simulink library "DBX_Control_lib"  (R2015a)
settings: Solver=ode45  SolverMode=SingleTasking  StartTime=0.0  StopTime=10.0  RelTol=1e-3
undefined symbols (not defined in the file): a, A_M, C_d0, CG, h_1, h_2, h_3, hp_1, kappa_Q, kappa_T, L_M, lambda_0_Q, lambda_0_T, m, Newton, Omega_TO, R, Raphson, rho, Rotation_sign, sigma, T_ctrl, T_sim, theta_0, theta_1, Throtle_TO, Throtle_TTO_vec, v_i0, v_i_adim, Vx_adim, Vz_adim
libraries: DBX_Control_lib x15, vrlib x7, DBX_model x2, qcatlib x1, simulink x1, XXCopter_Control x1
(part 2 of 2)

== system DBX_Control_lib/Ref Model and PI Controller/PI Controller ==
  y_c : Inport
  y_meas : Inport  Port=2
  Anti-windup signal : Inport  Port=3
  Int_reset : Inport  Port=4
  " " : Sum  Inputs=++-
  " 1" : Sum  Inputs=|++
  Add : Sum  Inputs=|+-
  Discrete-Time Integrator : DiscreteIntegrator  ExternalReset=either  InitialConditionSetting=State (most efficient)  SampleTime=T_ctrl
  K_a : Gain  Gain=K_a
  K_b : Gain  Gain=K_b
  f_c : Gain  Gain=f_c
  f_i*K_b : Gain  Gain=f_i*K_b
  y_des_dot : Outport
  wires:
  f_i*K_b/1 -> " 1"/1
  Add/1 -> f_i*K_b/1
  K_b/1 -> y_des_dot/1
  y_meas/1 -> " "/3, Add/2
  y_c/1 -> f_c/1, Add/1
  Discrete-Time Integrator/1 -> " "/2
  f_c/1 -> " "/1
  " "/1 -> K_b/1
  Anti-windup signal/1 -> K_a/1
  " 1"/1 -> Discrete-Time Integrator/1
  K_a/1 -> " 1"/2
  Int_reset/1 -> Discrete-Time Integrator/2

== system DBX_Control_lib/Ref Model and PI Controller/Reference Model ==
  y_ref : Inport
  y_i : Inport  Port=2
  Int_reset : Inport  Port=3
  Add : Sum  Inputs=|+-
  Discrete-Time Integrator : DiscreteIntegrator  ExternalReset=either  InitialConditionSource=external  InitialConditionSetting=State (most efficient)  SampleTime=T_ctrl
  K_ref : Gain  Gain=1/tau
  y_c_dot : Outport
  y_c : Outport  Port=2
  wires:
  y_ref/1 -> Add/1
  Add/1 -> K_ref/1
  K_ref/1 -> y_c_dot/1, Discrete-Time Integrator/1
  Discrete-Time Integrator/1 -> Add/2, y_c/1
  y_i/1 -> Discrete-Time Integrator/3
  Int_reset/1 -> Discrete-Time Integrator/2

== system DBX_Control_lib/Arm Dynamics/Aerodynamics Propeller DBX/2D vec norm1 ==
  v : Inport
  norm^2rm : Subsystem  TreatAsAtomicUnit=on
  sqrt : Sqrt  AlgorithmType=Newton-Raphson  SaturateOnIntegerOverflow=on
  norm(v) : Outport
  wires:
  v/1 -> norm^2rm/1(v)
  norm^2rm/1(norm(v)) -> sqrt/1
  sqrt/1 -> norm(v)/1

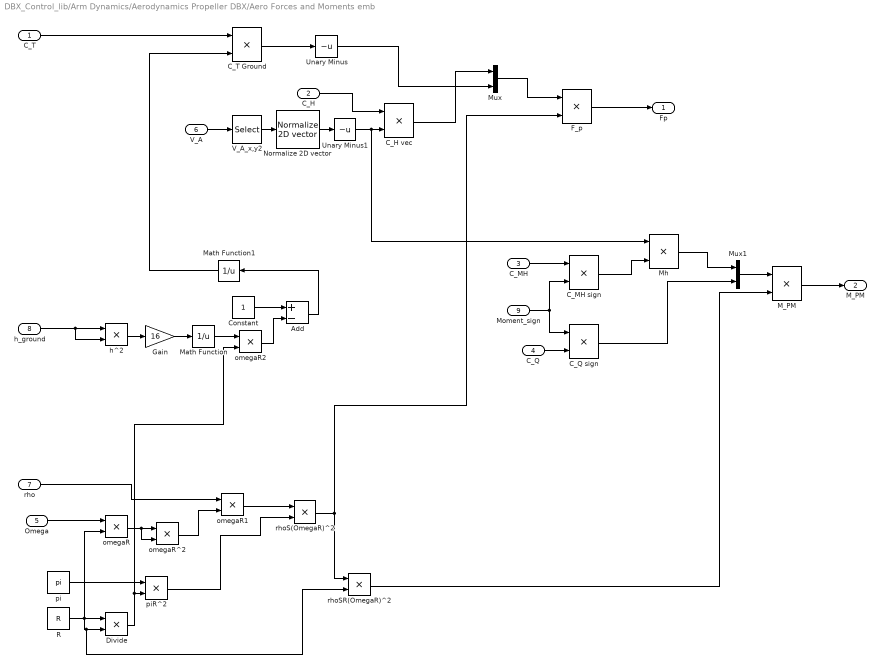
== system DBX_Control_lib/Arm Dynamics/Aerodynamics Propeller DBX/Aero Forces and Moments emb ==
  C_T : Inport
  C_H : Inport  Port=2
  C_MH : Inport  Port=3
  C_Q : Inport  Port=4
  Omega : Inport  Port=5
  V_A : Inport  Port=6
  rho : Inport  Port=7
  h_ground : Inport  Port=8
  Moment_sign : Inport  Port=9
  Add : Sum  Inputs=+-
  C_H vec : Product  Inputs=**
  C_MH sign : Product  Inputs=**
  C_Q sign : Product  Inputs=**
  C_T Ground : Product  Inputs=**
  Constant : Constant  OutDataTypeStr=single
  Divide : Product  Inputs=**
  F_p : Product  Inputs=**
  Gain : Gain  Gain=16  OutDataTypeStr=single
  M_PM : Product  Inputs=**
  Math Function : Math  Operator=reciprocal  SaturateOnIntegerOverflow=on
  Math Function1 : Math  Operator=reciprocal  SaturateOnIntegerOverflow=on
  Mh : Product  Inputs=**
  Mux : Mux  Inputs=[2,1]
  Mux1 : Mux  Inputs=[2,1]
  Normalize 2D vector : DBX_model/Normalize 2D vector
  R : Constant  Value=R  OutDataTypeStr=single
  Unary Minus : UnaryMinus
  Unary Minus1 : UnaryMinus
  V_A_x,y2 : Selector  IndexMode=Zero-based  InputPortWidth=3  Indices=[0,1]
  h^2 : Product  Inputs=**
  omegaR : Product  Inputs=**
  omegaR1 : Product  Inputs=**
  omegaR2 : Product  Inputs=**
  omegaR^2 : Product  Inputs=**
  pi : Constant  Value=pi  OutDataTypeStr=single
  piR^2 : Product  Inputs=**
  rhoS(OmegaR)^2 : Product  Inputs=**
  rhoSR(OmegaR)^2 : Product  Inputs=**
  Fp : Outport
  "M_PM " : Outport  Port=2
  wires:
  M_PM/1 -> "M_PM "/1
  rhoSR(OmegaR)^2/1 -> M_PM/2
  C_Q sign/1 -> Mux1/2
  C_Q/1 -> C_Q sign/2
  Mux1/1 -> M_PM/1
  F_p/1 -> Fp/1
  Mh/1 -> Mux1/1
  C_MH sign/1 -> Mh/2
  Moment_sign/1 -> C_Q sign/1, C_MH sign/2
  C_MH/1 -> C_MH sign/1
  rhoS(OmegaR)^2/1 -> F_p/2, rhoSR(OmegaR)^2/1
  Mux/1 -> F_p/1
  Unary Minus/1 -> Mux/2
  C_H vec/1 -> Mux/1
  C_H/1 -> C_H vec/1
  Unary Minus1/1 -> C_H vec/2, Mh/1
  Normalize 2D vector/1 -> Unary Minus1/1
  V_A/1 -> V_A_x,y2/1
  V_A_x,y2/1 -> Normalize 2D vector/1
  C_T Ground/1 -> Unary Minus/1
  Math Function1/1 -> C_T Ground/2
  Add/1 -> Math Function1/1
  omegaR2/1 -> Add/2
  Constant/1 -> Add/1
  Math Function/1 -> omegaR2/1
  Gain/1 -> Math Function/1
  h^2/1 -> Gain/1
  h_ground/1 -> h^2/1, h^2/2
  C_T/1 -> C_T Ground/1
  omegaR1/1 -> rhoS(OmegaR)^2/1
  piR^2/1 -> rhoS(OmegaR)^2/2
  omegaR^2/1 -> omegaR1/2
  omegaR/1 -> omegaR^2/1, omegaR^2/2
  rho/1 -> omegaR1/1
  Omega/1 -> omegaR/1
  Divide/1 -> piR^2/2, omegaR2/2
  pi/1 -> piR^2/1
  R/1 -> Divide/1, omegaR/2, Divide/2, rhoSR(OmegaR)^2/2

== system DBX_Control_lib/Arm Dynamics/Aerodynamics Propeller DBX/RAND_induced ==
  v_x_adim : Inport
  v_z_adim : Inport  Port=2
  Constant : Constant  OutDataTypeStr=single
  Divide : Product  Inputs=*/
  If : If  IfExpression=u1<=-2  ElseIfExpressions=u1>-2 & u1<0, u1 >= 0  ShowElse=off
  If Action Subsystem : Subsystem  TreatAsAtomicUnit=on
  If Action Subsystem1 : Subsystem  TreatAsAtomicUnit=on
  If Action Subsystem2 : Subsystem  TreatAsAtomicUnit=on
  Math Function : Math  Operator=square  SaturateOnIntegerOverflow=on
  Merge : Merge  Inputs=3
  Sqrt : Sqrt  SaturateOnIntegerOverflow=on
  Sum : Sum  Inputs=|++
  v_i_adim : Outport
  wires:
  Divide/1 -> v_i_adim/1
  Sqrt/1 -> Divide/2
  v_x_adim/1 -> Math Function/1, If/1
  Sum/1 -> Sqrt/1
  If/3 -> If Action Subsystem2/Action
  If/2 -> If Action Subsystem1/Action
  Constant/1 -> Sum/2
  Math Function/1 -> Sum/1
  v_z_adim/1 -> If Action Subsystem2/1(In1), If Action Subsystem1/1(v_z_adim), If Action Subsystem/1(v_z_adim)
  Merge/1 -> Divide/1
  If Action Subsystem2/1(Out1) -> Merge/3
  If Action Subsystem1/1(v_ia_adim) -> Merge/2
  If Action Subsystem/1(v_ia_adim) -> Merge/1
  If/1 -> If Action Subsystem/Action

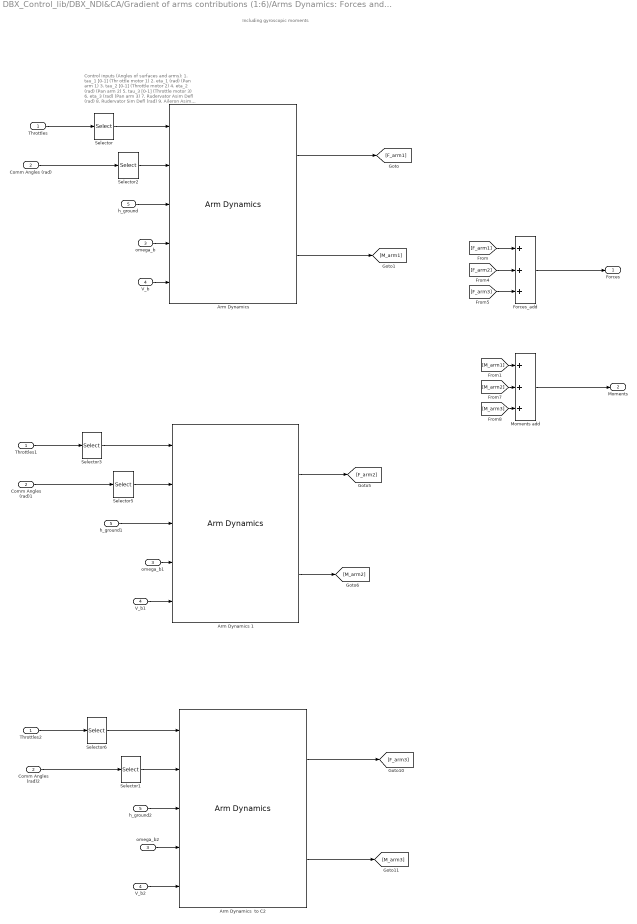
== system DBX_Control_lib/DBX_NDI&CA/Gradient of arms contributions (1:6)/Arms Dynamics: Forces and Moments ==
  note: Control inputs (Angles  of surfaces and arms):
      |
      | 1. tau_1 [0-1] (Thr ottle motor 1)
      | 2. eta_1 (rad)  (Pan arm 1)
      |
      | 3. tau_2 [0-1] (Throttle motor 2)
      | 4. eta_2 (rad)  (Pan arm 2)
      |
      | 5. tau_3 [0-1] (Throttle motor 3)
      | 6. eta_3 (rad)  (Pan arm  3)
      |
      | 7. Rudervator Asim Defl (rad)
      | 8. Rudervator Sim Defl (rad)
      | 9. Aileron Asim Defl (rad)
  note: Including gyroscopic moments
  Throttles : Inport
  Comm Angles (rad) : Inport  Port=2
  omega_b : Inport  Port=3
  V_b : Inport  Port=4
  h_ground : Inport  Port=5
  "Arm Dynamics " : DBX_Control_lib/Arm Dynamics  arm_num=1  Rot_sign=Rotation_sign(1)  Hub_pos=[1/3*L_M;-A_M/2;h_1]  h_p=hp_1
  Arm Dynamics  to C2 : DBX_Control_lib/Arm Dynamics  arm_num=3  Rot_sign=Rotation_sign(3)  Hub_pos=[-2/3*L_M;0;h_3]  h_p=hp_3
  Arm Dynamics 1 : DBX_Control_lib/Arm Dynamics  arm_num=2  Rot_sign=Rotation_sign(2)  Hub_pos=[1/3*L_M;A_M/2;h_2]  h_p=hp_2
  Comm Angles (rad)1 : InportShadow  Port=2
  Comm Angles (rad)2 : InportShadow  Port=2
  Forces_add : Sum  Inputs=+++
  Moments add : Sum  Inputs=+++
  Selector : Selector  IndexMode=Zero-based  InputPortWidth=3  Indices=0
  Selector1 : Selector  IndexMode=Zero-based  InputPortWidth=3  Indices=2
  Selector2 : Selector  InputPortWidth=3
  Selector3 : Selector  IndexMode=Zero-based  InputPortWidth=3
  Selector5 : Selector  InputPortWidth=3  Indices=2
  Selector6 : Selector  IndexMode=Zero-based  InputPortWidth=3  Indices=2
  Throttles1 : InportShadow
  Throttles2 : InportShadow
  V_b1 : InportShadow  Port=4
  V_b2 : InportShadow  Port=4
  h_ground1 : InportShadow  Port=5
  h_ground2 : InportShadow  Port=5
  omega_b1 : InportShadow  Port=3
  omega_b2 : InportShadow  Port=3
  Forces : Outport
  Moments : Outport  Port=2
  wires:
  V_b2/1 -> Arm Dynamics  to C2/5
  Arm Dynamics 1/2 -> [M_arm2]
  Throttles/1 -> Selector/1
  Selector/1 -> "Arm Dynamics "/1
  V_b/1 -> "Arm Dynamics "/5
  Forces_add/1 -> Forces/1
  Moments add/1 -> Moments/1
  h_ground/1 -> "Arm Dynamics "/3
  "Arm Dynamics "/1 -> [F_arm1]
  "Arm Dynamics "/2 -> [M_arm1]
  [F_arm1] -> Forces_add/1
  [M_arm1] -> Moments add/1
  omega_b/1 -> "Arm Dynamics "/4
  [F_arm2] -> Forces_add/2
  [F_arm3] -> Forces_add/3
  [M_arm3] -> Moments add/3
  [M_arm2] -> Moments add/2
  Selector2/1 -> "Arm Dynamics "/2
  Comm Angles (rad)/1 -> Selector2/1
  Throttles1/1 -> Selector3/1
  Selector3/1 -> Arm Dynamics 1/1
  V_b1/1 -> Arm Dynamics 1/5
  h_ground1/1 -> Arm Dynamics 1/3
  omega_b1/1 -> Arm Dynamics 1/4
  Selector5/1 -> Arm Dynamics 1/2
  Comm Angles (rad)1/1 -> Selector5/1
  Throttles2/1 -> Selector6/1
  Selector6/1 -> Arm Dynamics  to C2/1
  h_ground2/1 -> Arm Dynamics  to C2/3
  Arm Dynamics  to C2/1 -> [F_arm3]
  Arm Dynamics  to C2/2 -> [M_arm3]
  omega_b2/1 -> Arm Dynamics  to C2/4
  Selector1/1 -> Arm Dynamics  to C2/2
  Comm Angles (rad)2/1 -> Selector1/1
  Arm Dynamics 1/1 -> [F_arm2]

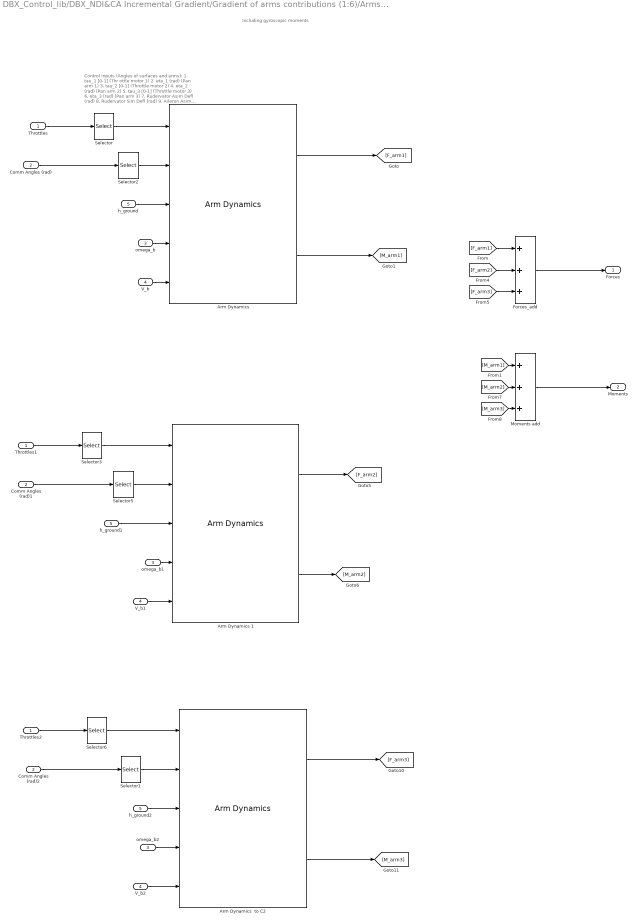
== system DBX_Control_lib/DBX_NDI&CA Incremental Gradient/Gradient of arms contributions (1:6)/Arms Dynamics: Forces and Moments ==
  note: Control inputs (Angles  of surfaces and arms):
      |
      | 1. tau_1 [0-1] (Thr ottle motor 1)
      | 2. eta_1 (rad)  (Pan arm 1)
      |
      | 3. tau_2 [0-1] (Throttle motor 2)
      | 4. eta_2 (rad)  (Pan arm 2)
      |
      | 5. tau_3 [0-1] (Throttle motor 3)
      | 6. eta_3 (rad)  (Pan arm  3)
      |
      | 7. Rudervator Asim Defl (rad)
      | 8. Rudervator Sim Defl (rad)
      | 9. Aileron Asim Defl (rad)
  note: Including gyroscopic moments
  Throttles : Inport
  Comm Angles (rad) : Inport  Port=2
  omega_b : Inport  Port=3
  V_b : Inport  Port=4
  h_ground : Inport  Port=5
  "Arm Dynamics " : DBX_Control_lib/Arm Dynamics  arm_num=1  Rot_sign=Rotation_sign(1)  Hub_pos=[1/3*L_M;-A_M/2;h_1]  h_p=hp_1
  Arm Dynamics  to C2 : DBX_Control_lib/Arm Dynamics  arm_num=3  Rot_sign=Rotation_sign(3)  Hub_pos=[-2/3*L_M;0;h_3]  h_p=hp_3
  Arm Dynamics 1 : DBX_Control_lib/Arm Dynamics  arm_num=2  Rot_sign=Rotation_sign(2)  Hub_pos=[1/3*L_M;A_M/2;h_2]  h_p=hp_2
  Comm Angles (rad)1 : InportShadow  Port=2
  Comm Angles (rad)2 : InportShadow  Port=2
  Forces_add : Sum  Inputs=+++
  Moments add : Sum  Inputs=+++
  Selector : Selector  IndexMode=Zero-based  InputPortWidth=3  Indices=0
  Selector1 : Selector  IndexMode=Zero-based  InputPortWidth=3  Indices=2
  Selector2 : Selector  InputPortWidth=3
  Selector3 : Selector  IndexMode=Zero-based  InputPortWidth=3
  Selector5 : Selector  InputPortWidth=3  Indices=2
  Selector6 : Selector  IndexMode=Zero-based  InputPortWidth=3  Indices=2
  Throttles1 : InportShadow
  Throttles2 : InportShadow
  V_b1 : InportShadow  Port=4
  V_b2 : InportShadow  Port=4
  h_ground1 : InportShadow  Port=5
  h_ground2 : InportShadow  Port=5
  omega_b1 : InportShadow  Port=3
  omega_b2 : InportShadow  Port=3
  Forces : Outport
  Moments : Outport  Port=2
  wires:
  V_b2/1 -> Arm Dynamics  to C2/5
  Arm Dynamics 1/2 -> [M_arm2]
  Throttles/1 -> Selector/1
  Selector/1 -> "Arm Dynamics "/1
  V_b/1 -> "Arm Dynamics "/5
  Forces_add/1 -> Forces/1
  Moments add/1 -> Moments/1
  h_ground/1 -> "Arm Dynamics "/3
  "Arm Dynamics "/1 -> [F_arm1]
  "Arm Dynamics "/2 -> [M_arm1]
  [F_arm1] -> Forces_add/1
  [M_arm1] -> Moments add/1
  omega_b/1 -> "Arm Dynamics "/4
  [F_arm2] -> Forces_add/2
  [F_arm3] -> Forces_add/3
  [M_arm3] -> Moments add/3
  [M_arm2] -> Moments add/2
  Selector2/1 -> "Arm Dynamics "/2
  Comm Angles (rad)/1 -> Selector2/1
  Throttles1/1 -> Selector3/1
  Selector3/1 -> Arm Dynamics 1/1
  V_b1/1 -> Arm Dynamics 1/5
  h_ground1/1 -> Arm Dynamics 1/3
  omega_b1/1 -> Arm Dynamics 1/4
  Selector5/1 -> Arm Dynamics 1/2
  Comm Angles (rad)1/1 -> Selector5/1
  Throttles2/1 -> Selector6/1
  Selector6/1 -> Arm Dynamics  to C2/1
  h_ground2/1 -> Arm Dynamics  to C2/3
  Arm Dynamics  to C2/1 -> [F_arm3]
  Arm Dynamics  to C2/2 -> [M_arm3]
  omega_b2/1 -> Arm Dynamics  to C2/4
  Selector1/1 -> Arm Dynamics  to C2/2
  Comm Angles (rad)2/1 -> Selector1/1
  Arm Dynamics 1/1 -> [F_arm2]

== system DBX_Control_lib/Normalize 4D vector/4D vec norm/norm^2rm ==
  v : Inport
  Demux : Demux
  Product{,1..3} (4 alike) : Product
  Sum : Sum  Inputs=4
  norm(v) : Outport
  wires:
  Product3/1 -> Sum/4
  Demux/4 -> Product3/1, Product3/2
  Product2/1 -> Sum/3
  Demux/3 -> Product2/1, Product2/2
  v/1 -> Demux/1
  Sum/1 -> norm(v)/1
  Product/1 -> Sum/1
  Product1/1 -> Sum/2
  Demux/1 -> Product/1, Product/2
  Demux/2 -> Product1/1, Product1/2

== system DBX_Control_lib/Arm Dynamics/Aerodynamics Propeller DBX/2D vec norm1/norm^2rm ==
  v : Inport
  Demux : Demux  Outputs=2
  Product : Product
  Product1 : Product
  Sum : Sum  Inputs=2
  norm(v) : Outport
  wires:
  Demux/1 -> Product/1, Product/2
  Product1/1 -> Sum/2
  Product/1 -> Sum/1
  Sum/1 -> norm(v)/1
  v/1 -> Demux/1
  Demux/2 -> Product1/2, Product1/1

== system DBX_Control_lib/Arm Dynamics/Aerodynamics Propeller DBX/RAND_induced/If Action Subsystem ==
  v_z_adim : Inport
  Action Port : ActionPort
  Subsystem : Subsystem
  v_ia_adim : Outport
  wires:
  v_z_adim/1 -> Subsystem/1(v_z_adim)
  Subsystem/1(v_ia_adim #1) -> v_ia_adim/1

== system DBX_Control_lib/Arm Dynamics/Aerodynamics Propeller DBX/RAND_induced/If Action Subsystem1 ==
  v_z_adim : Inport
  Action Port : ActionPort
  Subsystem1 : Subsystem
  v_ia_adim : Outport
  wires:
  v_z_adim/1 -> Subsystem1/1(v_z_adim)
  Subsystem1/1(v_ia_adim #2) -> v_ia_adim/1

== system DBX_Control_lib/Arm Dynamics/Aerodynamics Propeller DBX/RAND_induced/If Action Subsystem2 ==
  In1 : Inport
  Action Port : ActionPort
  Subsystem1 : Subsystem
  Out1 : Outport
  wires:
  In1/1 -> Subsystem1/1(v_z_adim)
  Subsystem1/1(v_ia_adim #3) -> Out1/1

== system DBX_Control_lib/Arm Dynamics/Aerodynamics Propeller DBX/RAND_induced/If Action Subsystem/Subsystem ==
  v_z_adim : Inport
  Constant1 : Constant  Value=4  OutDataTypeStr=single
  Gain : Gain  Gain=0.5  OutDataTypeStr=single
  Math Function : Math  Operator=square  SaturateOnIntegerOverflow=on
  Sqrt1 : Sqrt  SaturateOnIntegerOverflow=on
  Sum : Sum  Inputs=|++
  Sum1 : Sum  Inputs=|+-
  Unary Minus : UnaryMinus
  v_ia_adim #1 : Outport
  wires:
  Gain/1 -> Unary Minus/1
  Unary Minus/1 -> v_ia_adim #1/1
  Math Function/1 -> Sum1/1
  Constant1/1 -> Sum1/2
  Sum1/1 -> Sqrt1/1
  v_z_adim/1 -> Math Function/1, Sum/1
  Sum/1 -> Gain/1
  Sqrt1/1 -> Sum/2

== system DBX_Control_lib/Arm Dynamics/Aerodynamics Propeller DBX/RAND_induced/If Action Subsystem1/Subsystem1 ==
  v_z_adim : Inport
  25/12 : Constant  Value=2.083333333333334  OutDataTypeStr=single
  "3 " : Constant  Value=3  OutDataTypeStr=single
  7/6 : Constant  Value=1.166666666666667  OutDataTypeStr=single
  Constant1 : Constant  OutDataTypeStr=single
  Gain : Gain  Gain=0.5  OutDataTypeStr=single
  Math Function : Math  Operator=pow  SaturateOnIntegerOverflow=on
  Multiply : Product  Inputs=**
  Multiply1 : Product  Inputs=**
  Sum : Sum  Inputs=+-++
  v_ia_adim #2 : Outport
  wires:
  v_z_adim/1 -> Gain/1, Math Function/1, Multiply/1
  Sum/1 -> v_ia_adim #2/1
  25/12/1 -> Multiply/2
  Gain/1 -> Sum/2
  Constant1/1 -> Sum/1
  Multiply/1 -> Sum/3
  "3 "/1 -> Math Function/2
  Math Function/1 -> Multiply1/1
  7/6/1 -> Multiply1/2
  Multiply1/1 -> Sum/4

== system DBX_Control_lib/Arm Dynamics/Aerodynamics Propeller DBX/RAND_induced/If Action Subsystem2/Subsystem1 ==
  v_z_adim : Inport
  1 : Constant  Value=4  OutDataTypeStr=single
  Gain1 : Gain  Gain=0.5  OutDataTypeStr=single
  Math Function : Math  Operator=square  SaturateOnIntegerOverflow=on
  Sqrt : Sqrt  SaturateOnIntegerOverflow=on
  Sum : Sum  Inputs=|++
  Sum1 : Sum  Inputs=-+
  v_ia_adim #3 : Outport
  wires:
  Gain1/1 -> v_ia_adim #3/1
  Sum1/1 -> Gain1/1
  v_z_adim/1 -> Math Function/1, Sum1/1
  1/1 -> Sum/2
  Sum/1 -> Sqrt/1
  Math Function/1 -> Sum/1
  Sqrt/1 -> Sum1/2

== matlab function DBX_Control_lib/Arm Dynamics/Aerodynamics Propeller DBX/Prop Coefficients MOD ==
  data: lambda input; C_T output; mu input; C_H output; C_MH output; C_Q output; sigma parameter; C_d0 parameter; a parameter; theta_0 parameter; theta_1 parameter; lambda_0_T parameter; kappa_T parameter; lambda_0_Q parameter; kappa_Q parameter
function [C_T,C_H,C_MH,C_Q] = Aero_coeff_MOD(lambda,mu, sigma, C_d0, a, theta_0, theta_1,lambda_0_T,kappa_T,lambda_0_Q,kappa_Q)

C_T = sigma*a/4*(theta_0*(2/3+mu^2) +theta_1/2*(1+mu^2) -  kappa_T*(lambda-lambda_0_T)^2 );
C_Q =    +sigma*a/4*( 2/3*theta_0 -  kappa_Q*(lambda-lambda_0_Q)^2  + theta_1/2)*kappa_Q*(lambda-lambda_0_Q)^2 + sigma*C_d0/8*(1+mu^2);   % Always positive!!!


C_H= sigma*a/4*mu*lambda*(theta_0+theta_1/2) + sigma*C_d0/4*mu; 
C_MH= sigma*a/4*( 2/3*theta_0*mu-1/2*lambda*mu+theta_1*mu/2  );

== matlab function DBX_Control_lib/Arm Dynamics/Arms Kinematics DBX/DCM Arm ==
  data: arm_no input; eta input; T_Fb_FA output
function T_Fb_FA = DCM_Arm(arm_no,eta)
if arm_no==1 || arm_no==2
    T_Fb_FA = [ cos(eta),0,-sin(eta);
                    0,1,0;
                sin(eta),0,cos(eta)];
elseif arm_no==3 
    T_Fb_FA = [1,0,0;
                0,cos(eta),sin(eta);
                0,-sin(eta),cos(eta)];
else
    error('That is not right: Chose a right arm'); 
end

== matlab function DBX_Control_lib/DBX_NDI&CA Incremental Gradient/Get gradient ==
  data: index input; epsilon input; CA_Grad output; Perturb_evaluations input; CA_Grad_ant input
function CA_Grad  = Get_gradient(index, epsilon,Perturb_evaluations,CA_Grad_ant)

CA_Grad = CA_Grad_ant;

% Gradient of Arms: update
CA_Grad(:,index)= ( Perturb_evaluations(:,2)-Perturb_evaluations(:,1)  )./(epsilon);


% Eliminar componentes irrelevantes por el momento
CA_Grad(:,2)=zeros(6,1);
CA_Grad(:,4)=zeros(6,1);
CA_Grad(end,5)=0;
%% Add here the gradient of aerodynamics

% CA_Grad(4:6,7:10) ,,  B_adim*1/2*rho*S_w*TAS^2?? Cambiar esto esta mal


end

== matlab function DBX_Control_lib/Control allocator 4 coder/Embedded MATLAB Function ==
  data: v input; u output size=[9,1]; u_ant input; W input; ud input; B input; plim input; rlim input; T input size=1; Wv input; Wu input; gammma input size=1; imax input; W_out output size=[9,1]
function [u , W_out ] = qp_ca_WLS(v,u_ant,W,ud,B,plim,rlim,T,Wv,Wu, gammma,imax)


% Formulate as a regular QP problem: min ||Wu(u-ud)||

% Overall position limits
if isempty(rlim)
    umin = plim(:,1);
    umax = plim(:,2);
else
    umin = max(plim(:,1),u_ant+rlim(:,1)*T);
    umax = min(plim(:,2),u_ant+rlim(:,2)*T);
end

% Start with the last
u=u_ant;
W_out=W;

% Number of variables
m = length(umin);
%   Wu*(u-ud)
% Set default values of optional arguments
if nargin < 11
    imax = 100; % Heuristic value
    [k,m] = size(B);
    if nargin < 10, u = (umin+umax)/2; W = zeros(m,1); end
    if nargin < 8,  gammma = 1e6;       end
    if nargin < 7,  ud = zeros(m,1); end
    if nargin < 6,  Wu = eye(m);     end
    if nargin < 5,  Wv = eye(k);     end
end

gammma_sq = sqrt(gammma);
A = [gammma_sq*Wv*B ; Wu];
b = [gammma_sq*Wv*v ; Wu*ud];

% Initial residual.
d = b - A*u;
% Determine indeces of free variables.
i_free = zeros(size(W));
i_free = (W==0);

% Iterate until optimum is found or maximum number of iterations
% is reached.
for iter = 1:imax
    % ----------------------------------------
    %  Compute optimal perturbation vector p.
    % ----------------------------------------
    
    % Eliminate saturated variables.
    A_free = A(:,i_free);
    % Solve the reduced optimization problem for free variables.
    p_free = A_free\d;
    % Zero all perturbations corresponding to active constraints.
    p = zeros(m,1);
    % Insert perturbations from p_free into free the variables.
    p(i_free) = p_free;
    
    % ----------------------------
    %  Is the new point feasible?
    % ----------------------------
    
    u_opt = u + p;
    infeasible = (u_opt < umin) | (u_opt > umax);
    
    if ~any(infeasible(i_free))
        
        % ----------------------------
        %  Yes, check for optimality.
        % ----------------------------
        
        % Update point and residual.
        u = u_opt;
        d = d - A_free*p_free;
        % Compute Lagrangian multipliers.
        lambda = W.*(A'*d);
        % Are all lambda non-negative?
        if min(lambda) >= -eps
            % / ------------------------ \
            % | Optimum found, bail out. |
            % \ ------------------------ /
            return;
        end
        
        % --------------------------------------------------
        %  Optimum not found, remove one active constraint.
        % --------------------------------------------------
        
        % Remove constraint with most negative lambda from the
        % working set.
        [lambda_neg,i_neg] = min(lambda);
        W_out(i_neg) = 0;
        i_free(i_neg) = 1;
        
    else
        
        % ---------------------------------------
        %  No, find primary bounding constraint.
        % ---------------------------------------
        
        % Compute distances to the different boundaries. Since alpha < 1
        % is the maximum step length, initiate with ones.
        dist = ones(m,1);
        i_min = i_free & p<0;
        i_max = i_free & p>0;
        
        dist(i_min) = (umin(i_min) - u(i_min)) ./ p(i_min);
        dist(i_max) = (umax(i_max) - u(i_max)) ./ p(i_max);
        
        % Proportion of p to travel
        [alpha,i_alpha] = min(dist);
        % Update point and residual.
        u = u + alpha*p;
        d = d - A_free*alpha*p_free;
        
        % Add corresponding constraint to working set.
        W_out(i_alpha) = sign(p(i_alpha));
        i_free(i_alpha) = 0;
        
    end
    
    
end


end

== matlab function DBX_Control_lib/DBX_NDI&CA/Gravity Force and Moment ==
  data: q input; F_g_b output; M_g_b output; mass input; CG input; g parameter
function [F_g_b,M_g_b]   = Grav_Forces_and_Mom( q,mass,CG, g)

Prod=HamiltonProduct([q(1);-q(2);-q(3);-q(4)],HamiltonProduct([0;0;0;mass*g],[q(1);q(2);q(3);q(4)]) ); % q* . g .q

F_g_b= Prod(2:4);
M_g_b=cross(CG,F_g_b);


function Product= HamiltonProduct( a,b )

Product=[ a(1)*b(1)-a(2)*b(2)-a(3)*b(3)-a(4)*b(4) ; a(1)*b(2)+a(2)*b(1)+a(3)*b(4)-a(4)*b(3)  ; a(1)*b(3)-a(2)*b(4)+a(3)*b(1)+a(4)*b(2)  ; a(1)*b(4)+a(2)*b(3)-a(3)*b(2)+a(4)*b(1) ];

== matlab function DBX_Control_lib/DBX_NDI&CA Incremental Gradient/Gravity Force and Moment ==
  data: q input; F_g_b output; M_g_b output; mass input; CG input; g parameter
function [F_g_b,M_g_b]   = Grav_Forces_and_Mom( q,mass,CG, g)

Prod=HamiltonProduct([q(1);-q(2);-q(3);-q(4)],HamiltonProduct([0;0;0;mass*g],[q(1);q(2);q(3);q(4)]) ); % q* . g .q

F_g_b= Prod(2:4);
M_g_b=cross(CG,F_g_b);


function Product= HamiltonProduct( a,b )

Product=[ a(1)*b(1)-a(2)*b(2)-a(3)*b(3)-a(4)*b(4) ; a(1)*b(2)+a(2)*b(1)+a(3)*b(4)-a(4)*b(3)  ; a(1)*b(3)-a(2)*b(4)+a(3)*b(1)+a(4)*b(2)  ; a(1)*b(4)+a(2)*b(3)-a(3)*b(2)+a(4)*b(1) ];

== matlab function DBX_Control_lib/DBX_NDI&CA/Get gradient ==
  data: epsilon input; CA_Grad output; Perturb_evaluations input
function CA_Grad  = Get_gradient(epsilon,Perturb_evaluations)

CA_Grad = zeros(6,9);

% Gradient of Arms
for i=1:6
    CA_Grad(:,i)= ( Perturb_evaluations(:,2*i)-Perturb_evaluations(:,2*i-1)  )./(epsilon);
end

% Eliminar componentes irrelevantes por el momento
CA_Grad(:,2)=zeros(6,1);
CA_Grad(:,4)=zeros(6,1);
CA_Grad(end,5)=0;
%% Add here the gradient of aerodynamics

% CA_Grad(4:6,7:10) ,,  B_adim*1/2*rho*S_w*TAS^2?? Cambiar esto esta mal


end

== matlab function DBX_Control_lib/DBX_NDI&CA/Perturbations ==
  data: epsilon input; Ctrl_input input; Pert_Ctrl output
function Pert_Ctrl  = Perturbate_input(epsilon, Ctrl_input)
% The control input has a dimension of 6
% The gradient is computed with 2 evaluations, so the output vector has
% 2*6*6 components

Pert_Ctrl=zeros(2*6*6,1);

for i=1:6
    % Left
    tmp=Ctrl_input;
    tmp(i)=tmp(i)-epsilon;
    Pert_Ctrl( 1+2*(i-1)*6:(2*i-1)*6 ) = tmp;
    % Right
    tmp=Ctrl_input;
    tmp(i)=tmp(i)+epsilon;
    Pert_Ctrl( 1+(2*i-1)*6 :2*i*6 ) = tmp;
end






end
